simulink model "TP1_simu"  (R2023b)
settings: Solver=VariableStepAuto  StartTime=0.0  StopTime=10.0  RelTol=1e-3
values from neighbouring files (symbols this model uses):
  C1g = C1*k    [TP1.m]
  Dig = zpk(4/Ts, -4/Ts, -1)    [TP1.m]
  ue = 4    [TP1.m]
  x1e = 1    [TP1.m]
  x2e = 1    [TP1.m]
  x3e = 0    [TP1.m]
  ye = x2e    (= 1)    [TP1.m]
libraries: cstblocks x4
settings Model: Creator=manuh  LastModifiedBy=manuh

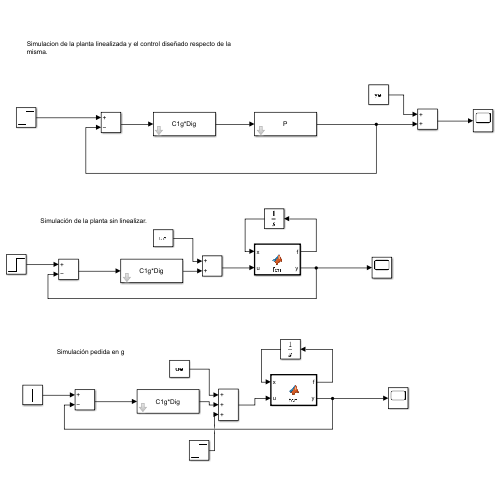
[thumbnail: Simulink's stored preview of the top-level diagram]
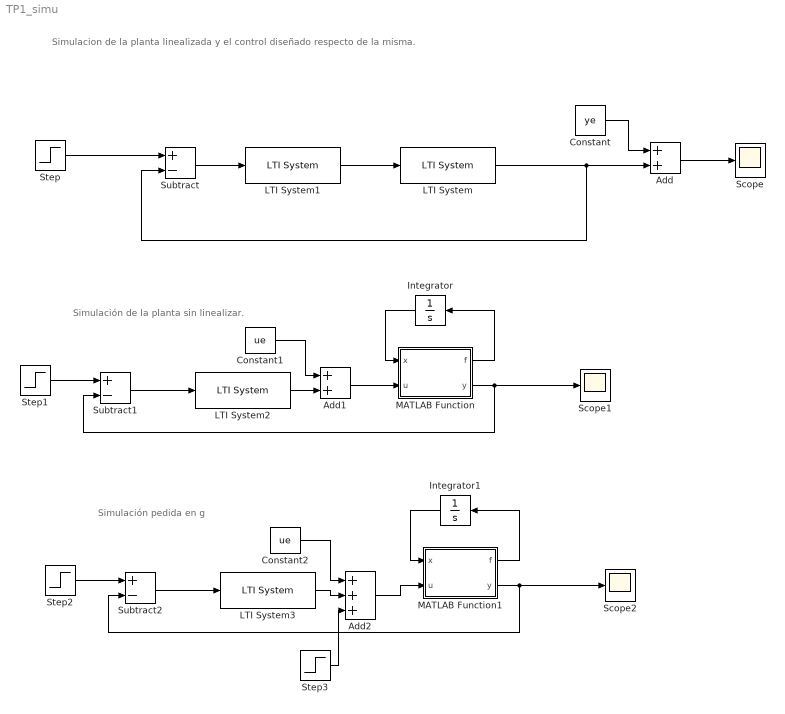
== system TP1_simu ==
  note: Simulación de la planta sin linealizar.
  note: Simulacion de la planta linealizada y el control diseñado respecto de la misma.
  note: Simulación pedida en g
  Add : Sum
  Add1 : Sum
  Add2 : Sum  Inputs=+++
  Constant : Constant  Value=ye
  Constant1 : Constant  Value=ue
  Constant2 : Constant  Value=ue
  Integrator : Integrator  InitialCondition=[x1e, x2e, x3e]
  Integrator1 : Integrator  InitialCondition=[x1e, x2e, x3e]
  LTI System : cstblocks/LTI System  sys=P  IC=[]  PadeOrder=0
  LTI System1 : cstblocks/LTI System  sys=C1g*Dig  IC=[]  PadeOrder=0
  LTI System2 : cstblocks/LTI System  sys=C1g*Dig  IC=[]  PadeOrder=0
  LTI System3 : cstblocks/LTI System  sys=C1g*Dig  IC=[]  PadeOrder=0
  MATLAB Function : MATLAB Function  TreatAsAtomicUnit=on
  MATLAB Function1 : MATLAB Function  TreatAsAtomicUnit=on
  Scope : Scope
  Scope1 : Scope
  Scope2 : Scope
  Step : Step  Time=2  After=0.05  SampleTime=0
  Step1 : Step  Time=2  Before=ye  After=ye+(ye*0.05)  SampleTime=0
  Step2 : Step  Time=2  Before=ye  After=ye+(ye*0.5)  SampleTime=0
  Step3 : Step  Time=6  After=ue*0.5  SampleTime=0
  Subtract : Sum  Inputs=+-
  Subtract1 : Sum  Inputs=+-
  Subtract2 : Sum  Inputs=+-
  wires:
  LTI System/1 -> Subtract/2, Add/2
  Subtract/1 -> LTI System1/1
  Step/1 -> Subtract/1
  LTI System1/1 -> LTI System/1
  Constant/1 -> Add/1
  Add/1 -> Scope/1
  Constant1/1 -> Add1/1
  LTI System2/1 -> Add1/2
  Add1/1 -> MATLAB Function/2(u)
  MATLAB Function/1(f) -> Integrator/1
  Integrator/1 -> MATLAB Function/1(x)
  Subtract1/1 -> LTI System2/1
  MATLAB Function/2(y) -> Scope1/1, Subtract1/2
  Step1/1 -> Subtract1/1
  Constant2/1 -> Add2/1
  MATLAB Function1/2(y) -> Scope2/1, Subtract2/2
  Integrator1/1 -> MATLAB Function1/1(x)
  Step2/1 -> Subtract2/1
  Add2/1 -> MATLAB Function1/2(u)
  Subtract2/1 -> LTI System3/1
  MATLAB Function1/1(f) -> Integrator1/1
  LTI System3/1 -> Add2/2
  Step3/1 -> Add2/3

== matlab function TP1_simu/MATLAB Function ==
  data: x input; f output; u input; y output
function [f,y] = fcn(x,u)
%Parámetros del problema
R=4;
L=1e-2;
m=0.1;
g=10;

% Definir funciones de derivadas (f)
f1=u/L-(R/L)*x(1);
f2=x(3);
f3=g-(x(1))/(x(2)*m);

f = [f1; f2; f3];

% Definir la salida y
y=x(2);

== matlab function TP1_simu/MATLAB Function1 ==
  data: x input; f output; u input; y output
function [f,y] = fcn(x,u)
%Parámetros del problema
R=4;
L=1e-2;
m=0.1;
g=10;

% Definir funciones de derivadas (f)
f1=u/L-(R/L)*x(1);
f2=x(3);
f3=g-(x(1))/(x(2)*m);

f = [f1; f2; f3];

% Definir la salida y
y=x(2);
